simulink library "FIN"  (R2016b)
settings: Solver=VariableStepAuto  StartTime=0.0  StopTime=10.0  RelTol=1e-3
undefined symbols (not defined in the file or in its folder): FIN
libraries: aerolibtransform2 x3, aerolibasang x1
settings Model: Creator=Andrew  LastModifiedBy=Andrew

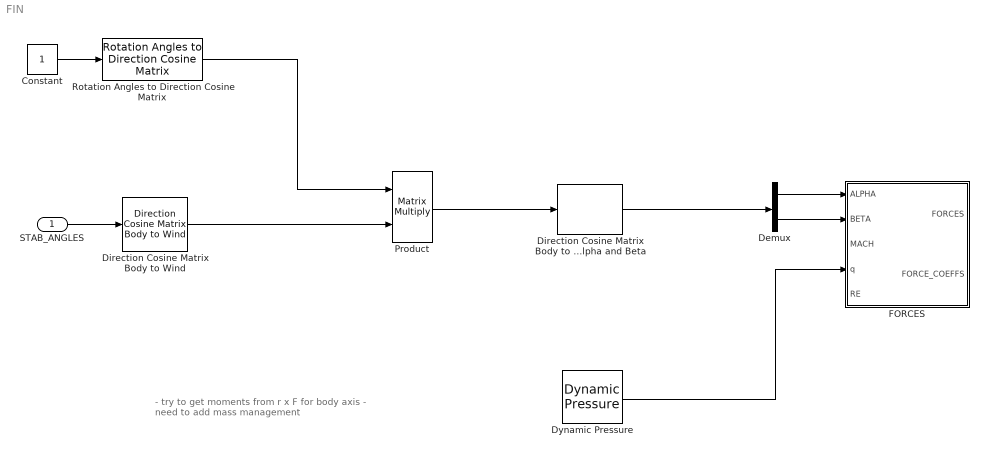
== system FIN ==
  note: - try to get moments from r x F for body axis
      | - need to add mass management
  STAB_ANGLES : Inport
  Constant : Constant
  Demux : Demux  Outputs=2
  Direction Cosine Matrix Body to Wind : aerolibtransform2/Direction Cosine Matrix Body to Wind
  Direction Cosine Matrix Body to Wind to Alpha and Beta : aerolibtransform2/Direction Cosine Matrix Body to Wind to Alpha and Beta
  Dynamic Pressure : aerolibasang/Dynamic Pressure
  FORCES : Subsystem
  Product : Product  Multiplication=Matrix(*)
  Rotation Angles to Direction Cosine Matrix : aerolibtransform2/Rotation Angles to Direction Cosine Matrix  rotationOrder=ZYX
  wires:
  Dynamic Pressure/1 -> FORCES/4(q)
  STAB_ANGLES/1 -> Direction Cosine Matrix Body to Wind/1
  Direction Cosine Matrix Body to Wind to Alpha and Beta/1 -> Demux/1
  Demux/1 -> FORCES/1(ALPHA)
  Demux/2 -> FORCES/2(BETA)
  Constant/1 -> Rotation Angles to Direction Cosine Matrix/1
  Product/1 -> Direction Cosine Matrix Body to Wind to Alpha and Beta/1
  Rotation Angles to Direction Cosine Matrix/1 -> Product/1
  Direction Cosine Matrix Body to Wind/1 -> Product/2

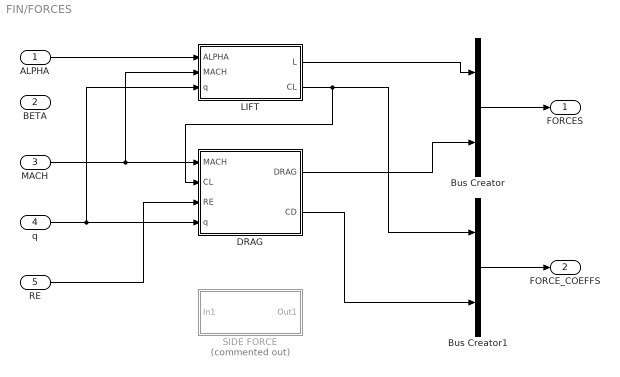
== system FIN/FORCES ==
  ALPHA : Inport
  BETA : Inport  Port=2
  MACH : Inport  Port=3
  q : Inport  Port=4
  RE : Inport  Port=5
  Bus Creator : BusCreator  Inputs=2
  Bus Creator1 : BusCreator  Inputs=2
  DRAG : Subsystem
  LIFT : Subsystem
  SIDE FORCE : Subsystem  Commented=on
  FORCES : Outport
  FORCE_COEFFS : Outport  Port=2
  wires:
  ALPHA/1 -> LIFT/1(ALPHA)
  Bus Creator/1 -> FORCES/1
  LIFT/1(L) -> Bus Creator/1
  Bus Creator1/1 -> FORCE_COEFFS/1
  LIFT/2(CL) -> DRAG/2(CL), Bus Creator1/1
  MACH/1 -> LIFT/2(MACH), DRAG/1(MACH)
  q/1 -> LIFT/3(q), DRAG/4(q)
  DRAG/1(DRAG) -> Bus Creator/2
  DRAG/2(CD) -> Bus Creator1/2
  RE/1 -> DRAG/3(RE)

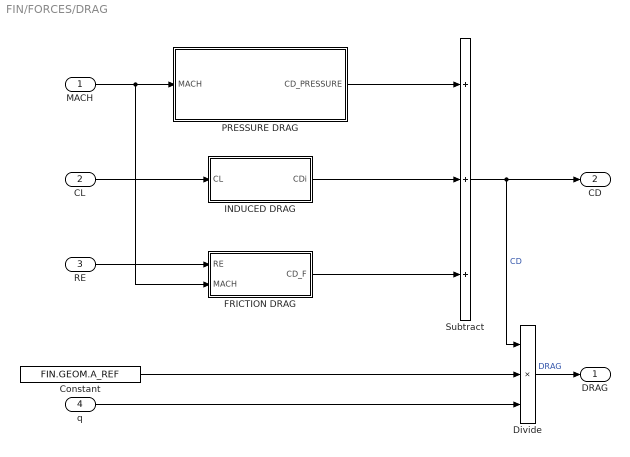
== system FIN/FORCES/DRAG ==
  MACH : Inport
  CL : Inport  Port=2
  RE : Inport  Port=3
  q : Inport  Port=4
  Constant : Constant  Value=FIN.GEOM.A_REF
  Divide : Product  Inputs=3
  FRICTION DRAG : Subsystem
  INDUCED DRAG : Subsystem
  PRESSURE DRAG : Subsystem
  Subtract : Sum  Inputs=+++
  DRAG : Outport
  CD : Outport  Port=2
  wires:
  PRESSURE DRAG/1(CD_PRESSURE) -> Subtract/1
  Subtract/1 -> Divide/1, CD/1  "CD"
  Divide/1 -> DRAG/1  "DRAG"
  q/1 -> Divide/3
  Constant/1 -> Divide/2
  FRICTION DRAG/1(CD_F) -> Subtract/3
  INDUCED DRAG/1(CDi) -> Subtract/2
  CL/1 -> INDUCED DRAG/1(CL)
  RE/1 -> FRICTION DRAG/1(RE)
  MACH/1 -> FRICTION DRAG/2(MACH), PRESSURE DRAG/1(MACH)

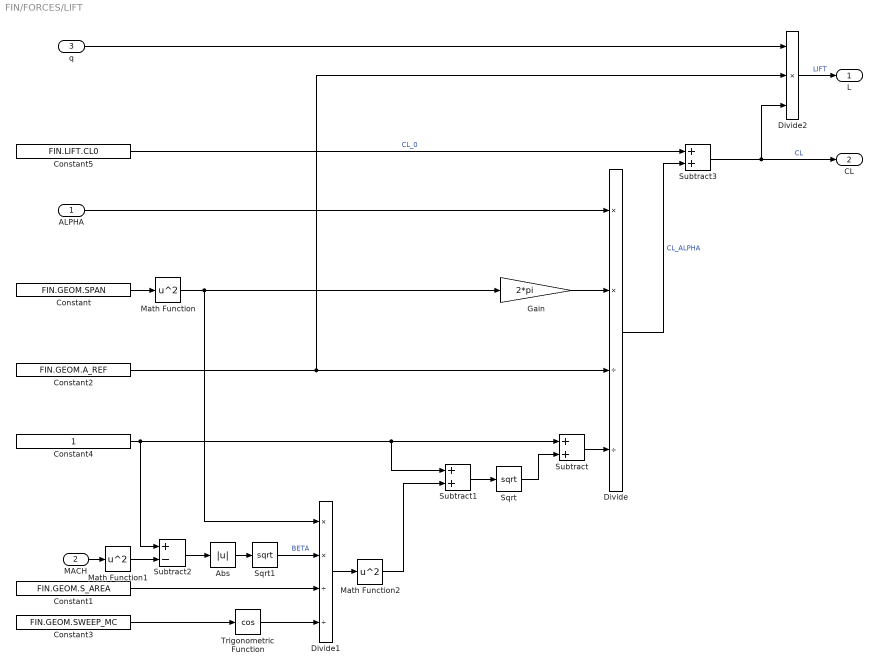
== system FIN/FORCES/LIFT ==
  ALPHA : Inport
  MACH : Inport  Port=2
  q : Inport  Port=3
  Abs : Abs
  Constant : Constant  Value=FIN.GEOM.SPAN
  Constant1 : Constant  Value=FIN.GEOM.S_AREA
  Constant2 : Constant  Value=FIN.GEOM.A_REF
  Constant3 : Constant  Value=FIN.GEOM.SWEEP_MC
  Constant4 : Constant
  Constant5 : Constant  Value=FIN.LIFT.CL0
  Divide : Product  Inputs=**//
  Divide1 : Product  Inputs=**//
  Divide2 : Product  Inputs=***
  Gain : Gain  Gain=2*pi
  Math Function : Math  Operator=square  SaturateOnIntegerOverflow=on
  Math Function1 : Math  Operator=square  SaturateOnIntegerOverflow=on
  Math Function2 : Math  Operator=square  SaturateOnIntegerOverflow=on
  Sqrt : Sqrt  SaturateOnIntegerOverflow=on
  Sqrt1 : Sqrt  SaturateOnIntegerOverflow=on
  Subtract : Sum
  Subtract1 : Sum
  Subtract2 : Sum  Inputs=+-
  Subtract3 : Sum
  Trigonometric Function : Trigonometry  Operator=cos
  L : Outport
  CL : Outport  Port=2
  wires:
  Constant/1 -> Math Function/1
  Math Function/1 -> Divide1/1, Gain/1
  Constant4/1 -> Subtract1/1, Subtract/1, Subtract2/1
  Sqrt/1 -> Subtract/2
  Subtract1/1 -> Sqrt/1
  Constant1/1 -> Divide1/3
  Constant3/1 -> Trigonometric Function/1
  Trigonometric Function/1 -> Divide1/4
  MACH/1 -> Math Function1/1
  Abs/1 -> Sqrt1/1
  Divide1/1 -> Math Function2/1
  Math Function2/1 -> Subtract1/2
  Subtract2/1 -> Abs/1
  Math Function1/1 -> Subtract2/2
  Sqrt1/1 -> Divide1/2  "BETA"
  Subtract/1 -> Divide/4
  Constant2/1 -> Divide2/2, Divide/3
  Gain/1 -> Divide/2
  ALPHA/1 -> Divide/1
  Constant5/1 -> Subtract3/1  "CL_0"
  Divide/1 -> Subtract3/2  "CL_ALPHA"
  Subtract3/1 -> CL/1, Divide2/3  "CL"
  Divide2/1 -> L/1  "LIFT"
  q/1 -> Divide2/1

== system FIN/FORCES/SIDE FORCE ==
  In1 : Inport
  Out1 : Outport
  wires:
  In1/1 -> Out1/1

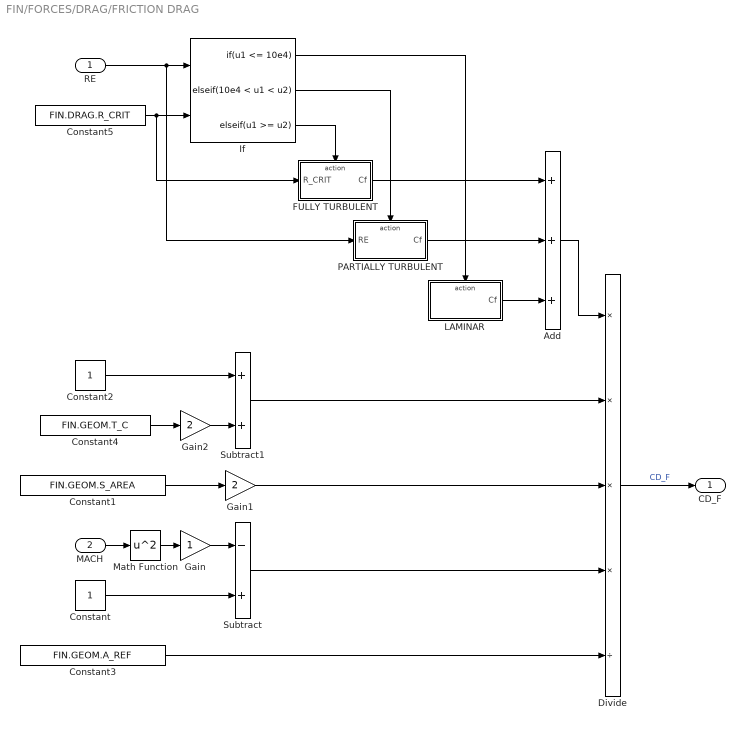
== system FIN/FORCES/DRAG/FRICTION DRAG ==
  RE : Inport
  MACH : Inport  Port=2
  Add : Sum  Inputs=+++
  Constant : Constant
  Constant1 : Constant  Value=FIN.GEOM.S_AREA
  Constant2 : Constant
  Constant3 : Constant  Value=FIN.GEOM.A_REF
  Constant4 : Constant  Value=FIN.GEOM.T_C
  Constant5 : Constant  Value=FIN.DRAG.R_CRIT
  Divide : Product  Inputs=****/
  FULLY TURBULENT : Subsystem  TreatAsAtomicUnit=on
  Gain : Gain
  Gain1 : Gain  Gain=2
  Gain2 : Gain  Gain=2
  If : If  NumInputs=2  IfExpression=u1 <= 10e4  ElseIfExpressions=10e4 < u1 < u2, u1 >= u2  ShowElse=off
  LAMINAR : Subsystem  TreatAsAtomicUnit=on
  Math Function : Math  Operator=square  SaturateOnIntegerOverflow=on
  PARTIALLY TURBULENT : Subsystem  TreatAsAtomicUnit=on
  Subtract : Sum  Inputs=-+
  Subtract1 : Sum
  CD_F : Outport
  wires:
  Divide/1 -> CD_F/1  "CD_F"
  MACH/1 -> Math Function/1
  Math Function/1 -> Gain/1
  Gain/1 -> Subtract/1
  Constant/1 -> Subtract/2
  Subtract/1 -> Divide/4
  Constant1/1 -> Gain1/1
  Gain1/1 -> Divide/3
  Subtract1/1 -> Divide/2
  Constant2/1 -> Subtract1/1
  Constant4/1 -> Gain2/1
  Gain2/1 -> Subtract1/2
  Constant3/1 -> Divide/5
  If/3 -> FULLY TURBULENT/Action
  If/2 -> PARTIALLY TURBULENT/Action
  If/1 -> LAMINAR/Action
  Constant5/1 -> FULLY TURBULENT/1(R_CRIT), If/2
  Add/1 -> Divide/1
  FULLY TURBULENT/1(Cf) -> Add/1
  LAMINAR/1(Cf) -> Add/3
  PARTIALLY TURBULENT/1(Cf) -> Add/2
  RE/1 -> PARTIALLY TURBULENT/1(RE), If/1

== system FIN/FORCES/DRAG/INDUCED DRAG ==
  CL : Inport
  Constant : Constant  Value=FIN.DRAG.EFF
  Constant1 : Constant  Value=FIN.GEOM.AR
  Divide : Product  Inputs=*//
  Gain : Gain  Gain=pi
  Math Function : Math  Operator=square  SaturateOnIntegerOverflow=on
  CDi : Outport
  wires:
  CL/1 -> Math Function/1
  Divide/1 -> CDi/1  "CDi"
  Math Function/1 -> Divide/1
  Constant/1 -> Gain/1
  Constant1/1 -> Divide/3
  Gain/1 -> Divide/2

== system FIN/FORCES/DRAG/PRESSURE DRAG ==
  MACH : Inport
  Add : Sum
  Leading Edge : Subsystem
  Trailing Edge : Subsystem
  CD_PRESSURE : Outport
  wires:
  Add/1 -> CD_PRESSURE/1
  Leading Edge/1(CD_FIN_LE) -> Add/1
  MACH/1 -> Trailing Edge/1(MACH), Leading Edge/1(MACH)
  Trailing Edge/1(CD_FIN_TE) -> Add/2

== system FIN/FORCES/DRAG/FRICTION DRAG/FULLY TURBULENT ==
  R_CRIT : Inport
  Action Port : ActionPort  ActionType=elseif
  Constant : Constant  Value=0.2/(-1.039)
  Gain : Gain  Gain=1/51
  Gain1 : Gain  Gain=0.032
  Math Function : Math  Operator=pow  SaturateOnIntegerOverflow=on
  Cf : Outport
  wires:
  R_CRIT/1 -> Gain/1
  Gain/1 -> Math Function/1
  Constant/1 -> Math Function/2
  Math Function/1 -> Gain1/1
  Gain1/1 -> Cf/1

== system FIN/FORCES/DRAG/FRICTION DRAG/LAMINAR ==
  Action Port : ActionPort  ActionType=then
  Constant : Constant  Value=1.48e-2
  Cf : Outport
  wires:
  Constant/1 -> Cf/1

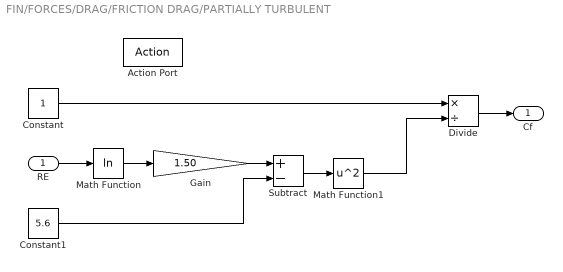
== system FIN/FORCES/DRAG/FRICTION DRAG/PARTIALLY TURBULENT ==
  RE : Inport
  Action Port : ActionPort  ActionType=elseif
  Constant : Constant
  Constant1 : Constant  Value=5.6
  Divide : Product  Inputs=*/
  Gain : Gain  Gain=1.50
  Math Function : Math  Operator=log  SaturateOnIntegerOverflow=on
  Math Function1 : Math  Operator=square  SaturateOnIntegerOverflow=on
  Subtract : Sum  Inputs=+-
  Cf : Outport
  wires:
  Constant/1 -> Divide/1
  Divide/1 -> Cf/1
  RE/1 -> Math Function/1
  Gain/1 -> Subtract/1
  Math Function/1 -> Gain/1
  Subtract/1 -> Math Function1/1
  Math Function1/1 -> Divide/2
  Constant1/1 -> Subtract/2

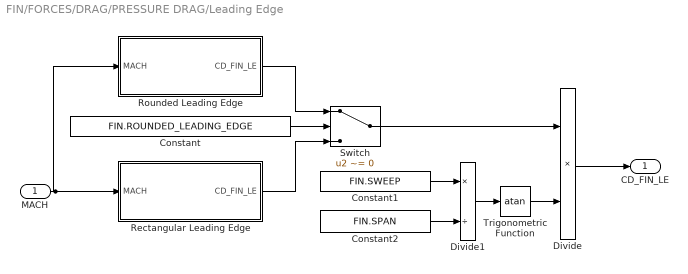
== system FIN/FORCES/DRAG/PRESSURE DRAG/Leading Edge ==
  MACH : Inport
  Constant : Constant  Value=FIN.ROUNDED_LEADING_EDGE
  Constant1 : Constant  Value=FIN.SWEEP
  Constant2 : Constant  Value=FIN.SPAN
  Divide : Product  Inputs=**
  Divide1 : Product  Inputs=*/
  Rectangular Leading Edge : Subsystem
  Rounded Leading Edge : Subsystem
  Switch : Switch  Criteria=u2 ~= 0
  Trigonometric Function : Trigonometry  Operator=atan
  CD_FIN_LE : Outport
  wires:
  Divide/1 -> CD_FIN_LE/1
  MACH/1 -> Rectangular Leading Edge/1(MACH), Rounded Leading Edge/1(MACH)
  Divide1/1 -> Trigonometric Function/1
  Trigonometric Function/1 -> Divide/2
  Switch/1 -> Divide/1
  Constant1/1 -> Divide1/1
  Constant2/1 -> Divide1/2
  Constant/1 -> Switch/2
  Rectangular Leading Edge/1(CD_FIN_LE) -> Switch/3
  Rounded Leading Edge/1(CD_FIN_LE) -> Switch/1

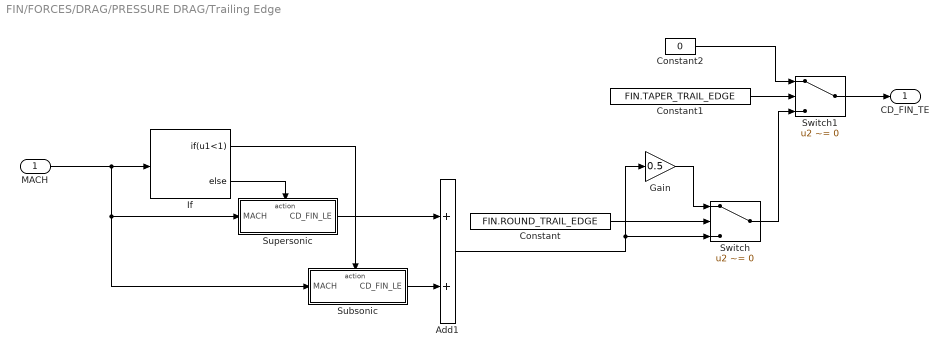
== system FIN/FORCES/DRAG/PRESSURE DRAG/Trailing Edge ==
  MACH : Inport
  Add1 : Sum
  Constant : Constant  Value=FIN.ROUND_TRAIL_EDGE
  Constant1 : Constant  Value=FIN.TAPER_TRAIL_EDGE
  Constant2 : Constant  Value=0
  Gain : Gain  Gain=0.5
  If : If  IfExpression=u1<1
  Subsonic : Subsystem  TreatAsAtomicUnit=on
  Supersonic : Subsystem  TreatAsAtomicUnit=on
  Switch : Switch  Criteria=u2 ~= 0
  Switch1 : Switch  Criteria=u2 ~= 0
  CD_FIN_TE : Outport
  wires:
  Constant2/1 -> Switch1/1
  Constant1/1 -> Switch1/2
  Switch1/1 -> CD_FIN_TE/1
  Switch/1 -> Switch1/3
  Gain/1 -> Switch/1
  Constant/1 -> Switch/2
  Add1/1 -> Switch/3, Gain/1
  MACH/1 -> If/1, Subsonic/1(MACH), Supersonic/1(MACH)
  Supersonic/1(CD_FIN_LE) -> Add1/1
  Subsonic/1(CD_FIN_LE) -> Add1/2
  If/1 -> Subsonic/Action
  If/2 -> Supersonic/Action

== system FIN/FORCES/DRAG/PRESSURE DRAG/Leading Edge/Rectangular Leading Edge ==
  MACH : Inport
  Add1 : Sum
  If : If  IfExpression=u1<1
  Subsonic : Subsystem  TreatAsAtomicUnit=on
  Supersonic : Subsystem  TreatAsAtomicUnit=on
  CD_FIN_LE : Outport
  wires:
  Add1/1 -> CD_FIN_LE/1
  If/2 -> Supersonic/Action
  If/1 -> Subsonic/Action
  Subsonic/1(CD_FIN_LE) -> Add1/2
  Supersonic/1(CD_FIN_LE) -> Add1/1
  MACH/1 -> Supersonic/1(MACH), Subsonic/1(MACH), If/1

== system FIN/FORCES/DRAG/PRESSURE DRAG/Leading Edge/Rounded Leading Edge ==
  MACH : Inport
  Add1 : Sum  Inputs=+++
  If : If  IfExpression=u1<0.9  ElseIfExpressions=u1>1
  Subsonic : Subsystem  TreatAsAtomicUnit=on
  Supersonic : Subsystem  TreatAsAtomicUnit=on
  Transonic : Subsystem  TreatAsAtomicUnit=on
  CD_FIN_LE : Outport
  wires:
  MACH/1 -> If/1, Subsonic/1(MACH), Supersonic/1(MACH), Transonic/1(MACH)
  Supersonic/1(CD_FIN_LE) -> Add1/2
  Transonic/1(CD_FIN_LE) -> Add1/1
  Subsonic/1(CD_FIN_LE) -> Add1/3
  If/2 -> Supersonic/Action
  If/1 -> Subsonic/Action
  If/3 -> Transonic/Action
  Add1/1 -> CD_FIN_LE/1

== system FIN/FORCES/DRAG/PRESSURE DRAG/Trailing Edge/Subsonic ==
  note: CD_LE = 1 + M^2/4 + M^4 / 40
  MACH : Inport
  Action Port : ActionPort
  Constant : Constant  Value=0.12
  Gain : Gain  Gain=0.13
  Math Function : Math  Operator=square  SaturateOnIntegerOverflow=on
  Subtract : Sum
  CD_FIN_LE : Outport
  wires:
  Constant/1 -> Subtract/2
  Math Function/1 -> Gain/1
  MACH/1 -> Math Function/1
  Subtract/1 -> CD_FIN_LE/1
  Gain/1 -> Subtract/1

== system FIN/FORCES/DRAG/PRESSURE DRAG/Trailing Edge/Supersonic ==
  MACH : Inport
  Action Port : ActionPort
  Gain : Gain  Gain=0.25
  Math Function : Math  Operator=reciprocal  SaturateOnIntegerOverflow=on
  CD_FIN_LE : Outport
  wires:
  Gain/1 -> CD_FIN_LE/1
  MACH/1 -> Math Function/1
  Math Function/1 -> Gain/1

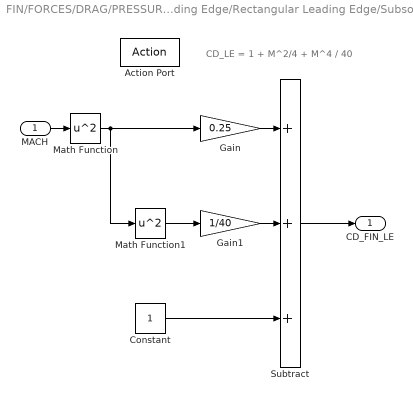
== system FIN/FORCES/DRAG/PRESSURE DRAG/Leading Edge/Rectangular Leading Edge/Subsonic ==
  note: CD_LE = 1 + M^2/4 + M^4 / 40
  MACH : Inport
  Action Port : ActionPort
  Constant : Constant
  Gain : Gain  Gain=0.25
  Gain1 : Gain  Gain=1/40
  Math Function : Math  Operator=square  SaturateOnIntegerOverflow=on
  Math Function1 : Math  Operator=square  SaturateOnIntegerOverflow=on
  Subtract : Sum  Inputs=+++
  CD_FIN_LE : Outport
  wires:
  Constant/1 -> Subtract/3
  Gain1/1 -> Subtract/2
  Math Function1/1 -> Gain1/1
  Gain/1 -> Subtract/1
  Subtract/1 -> CD_FIN_LE/1
  MACH/1 -> Math Function/1
  Math Function/1 -> Math Function1/1, Gain/1

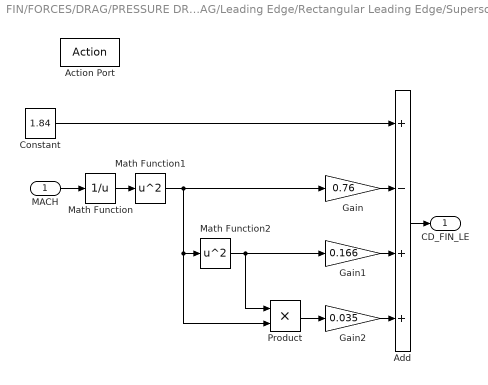
== system FIN/FORCES/DRAG/PRESSURE DRAG/Leading Edge/Rectangular Leading Edge/Supersonic ==
  MACH : Inport
  Action Port : ActionPort
  Add : Sum  Inputs=+-++
  Constant : Constant  Value=1.84
  Gain : Gain  Gain=0.76
  Gain1 : Gain  Gain=0.166
  Gain2 : Gain  Gain=0.035
  Math Function : Math  Operator=reciprocal  SaturateOnIntegerOverflow=on
  Math Function1 : Math  Operator=square  SaturateOnIntegerOverflow=on
  Math Function2 : Math  Operator=square  SaturateOnIntegerOverflow=on
  Product : Product
  CD_FIN_LE : Outport
  wires:
  Gain2/1 -> Add/4
  Gain1/1 -> Add/3
  Product/1 -> Gain2/1
  Math Function1/1 -> Gain/1, Product/2, Math Function2/1
  Math Function2/1 -> Product/1, Gain1/1
  Math Function/1 -> Math Function1/1
  MACH/1 -> Math Function/1
  Add/1 -> CD_FIN_LE/1
  Constant/1 -> Add/1
  Gain/1 -> Add/2

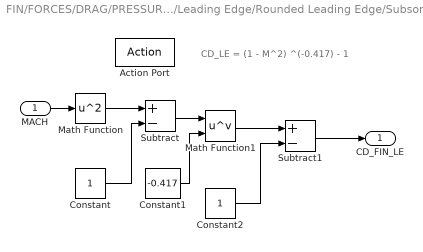
== system FIN/FORCES/DRAG/PRESSURE DRAG/Leading Edge/Rounded Leading Edge/Subsonic ==
  note: CD_LE = (1 - M^2) ^(-0.417) - 1
  MACH : Inport
  Action Port : ActionPort
  Constant : Constant
  Constant1 : Constant  Value=-0.417
  Constant2 : Constant
  Math Function : Math  Operator=square  SaturateOnIntegerOverflow=on
  Math Function1 : Math  Operator=pow  SaturateOnIntegerOverflow=on
  Subtract : Sum  Inputs=+-
  Subtract1 : Sum  Inputs=+-
  CD_FIN_LE : Outport
  wires:
  Subtract1/1 -> CD_FIN_LE/1
  Constant2/1 -> Subtract1/2
  Math Function1/1 -> Subtract1/1
  Constant1/1 -> Math Function1/2
  Subtract/1 -> Math Function1/1
  Constant/1 -> Subtract/2
  Math Function/1 -> Subtract/1
  MACH/1 -> Math Function/1

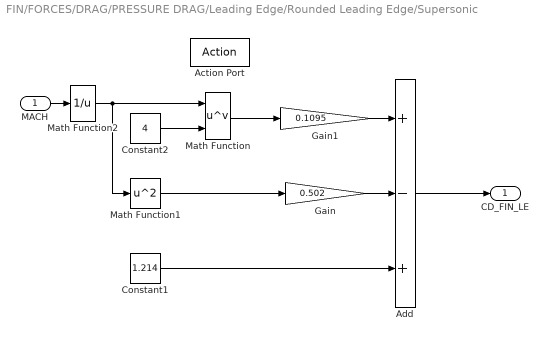
== system FIN/FORCES/DRAG/PRESSURE DRAG/Leading Edge/Rounded Leading Edge/Supersonic ==
  MACH : Inport
  Action Port : ActionPort
  Add : Sum  Inputs=+-+
  Constant1 : Constant  Value=1.214
  Constant2 : Constant  Value=4
  Gain : Gain  Gain=0.502
  Gain1 : Gain  Gain=0.1095
  Math Function : Math  Operator=pow  SaturateOnIntegerOverflow=on
  Math Function1 : Math  Operator=square  SaturateOnIntegerOverflow=on
  Math Function2 : Math  Operator=reciprocal  SaturateOnIntegerOverflow=on
  CD_FIN_LE : Outport
  wires:
  Gain1/1 -> Add/1
  Math Function/1 -> Gain1/1
  Add/1 -> CD_FIN_LE/1
  Constant2/1 -> Math Function/2
  Gain/1 -> Add/2
  Math Function1/1 -> Gain/1
  Math Function2/1 -> Math Function/1, Math Function1/1
  MACH/1 -> Math Function2/1
  Constant1/1 -> Add/3

== system FIN/FORCES/DRAG/PRESSURE DRAG/Leading Edge/Rounded Leading Edge/Transonic ==
  MACH : Inport
  Action Port : ActionPort
  Add : Sum  Inputs=-+
  Add1 : Sum  Inputs=+-
  Constant : Constant
  Constant1 : Constant  Value=0.9
  Gain : Gain  Gain=1.785
  CD_FIN_LE : Outport
  wires:
  Gain/1 -> Add/2
  Add1/1 -> Gain/1
  Constant1/1 -> Add1/2
  MACH/1 -> Add1/1
  Constant/1 -> Add/1
  Add/1 -> CD_FIN_LE/1
